simulink model "actuator_control"  (R2016b)
settings: configuration reference "Configuration4khz" (kept outside this file)
values from neighbouring files (symbols this model uses):
  sample_time = 0.0005    [ElmoIncremental.m]
undefined symbols (not defined in the file or in its folder): A_kalman_sea_swing_back, A_kalman_sea_swing_front, A_kalman_swing_load, A_lpf_1to4, A_lpf_dtau, A_lpf_sea_kalman_velocities, B1_lpf_1to4, B1_lpf_dtau, B1_lpf_sea_kalman_velocities, B2_lpf_1to4, B2_lpf_dtau, B2_lpf_sea_kalman_velocities, B_kalman_sea_swing_back, B_kalman_sea_swing_front, B_kalman_swing_load, C_kalman_sea_swing, C_kalman_swing_load, DiscIntNeverNeededParam, Discrete, elmo_sample_time, fdesignblkfcn, gcbh, initial_dx_estimate, j_segments, k_sea_low, kalman_load_to_deflect_transmission, lateral_motor_efficiency, LEG_MTR_GEAR_RATIO, P0_kalman_sea_swing, P0_kalman_swing_load, Q_kalman_load_torque, Q_kalman_rotor_torque, Q_kalman_trunk_torque, R_kalman_absolute_fail, R_kalman_absolute_normal, R_kalman_incremental_loaded, R_kalman_incremental_unloaded, sea_kalman_sample_time, swing_collision_damping_rate, Time
libraries: simulink x17, ctrlSharedLib x8, dsparch4 x5, dspfdesign x1
(part 3 of 3)

== matlab function actuator_control/SEA Controller (Velocity Based)/Nonlinear Spring Deflection ==
  data: deflections output; tau_sea input
function deflections   = SeaSpringDeflection( tau_sea )
     deflections = SeaSpringDeflection( tau_sea );
end

== matlab function actuator_control/Misc/Load Motion Disturbance Observer (Swing) Error-Proportional - 2nd order ==
  data: reset input; spring_torques input; d_hat_tp1 output size=[1 4]; positions input; velocities input; j_segments parameter; sample_time parameter
function d_hat_tp1  = disturbance_observer(reset, spring_torques, positions, velocities, j_segments, sample_time)

    order = 2;
    L = 2*2.^[1:order+1] .* factorial(order+1)./(factorial(order+1-(1:(order+1))).*factorial(1:order+1));
    N = 4;
    
    persistent z_t d_hat_t integral_term;
    if isempty(z_t)
        z_t = zeros(1,N);
        d_hat_t = zeros(1,N);
        integral_term = zeros(order,N);
    end
    
    for i=1:N
        if reset(i)
            z_t(i) = 0;
            d_hat_t(i) = 0;
            integral_term(:,i) = 0;
        end
    end
   
    % Define system
    A_d = [1, sample_time; 0, 1];
    Bu_d = [zeros(1,N); sample_time./j_segments];
    A_c = [0 1; 0 0];
    Bu_c = [zeros(1,N); 1./j_segments];
    Bd_c = [zeros(1,N); 1./j_segments];
    x = [positions'; velocities'];
    u = spring_torques;
 
    % Estimate disturbances
    z_tp1 = zeros(1,N);
    x_tp1 = zeros(2,N);
    d_hat_tp1 = zeros(1,N);
    for i=1:N
        z_tp1(i) = z_t(i) + sample_time*(pinv(Bd_c(:,i))*(A_c*x(:,i) + Bu_c(:,i)*u(i)) + d_hat_t(i));
        x_tp1(:,i) = A_d*x(:,i) + Bu_d(:,i)*u(i);
        integral_term(1,i) = integral_term(1,i) + sample_time*(pinv(Bd_c(:,i))*x_tp1(:,i) - z_tp1(i));
        for j=2:order
            integral_term(j,i) = integral_term(j,i) + sample_time*integral_term(j-1,i);
        end
        d_hat_tp1(i) = L*[(pinv(Bd_c(:,i))*x_tp1(:,i) - z_tp1(i)); integral_term(:,i)];
        d_hat_t(i) = d_hat_tp1(i);
        z_t(i) = z_tp1(i);
    end
    
end
